simulink model "startSensCompEnv"  (R2021a)
settings: Solver=VariableStepAuto  StartTime=0.0  StopTime=10.0  RelTol=1e-3
undefined symbols (not defined in the file): CubeSatTimeStep, IAU, initCond, km, s, vehicle
libraries: dspmathops x6, sharedtransform x3, aerolibtransform2 x1, aerolibconvert2 x1, aerolibutil x1, aerolibcelestial x1
settings Model: Creator=noraw  LastModifiedBy=noraw

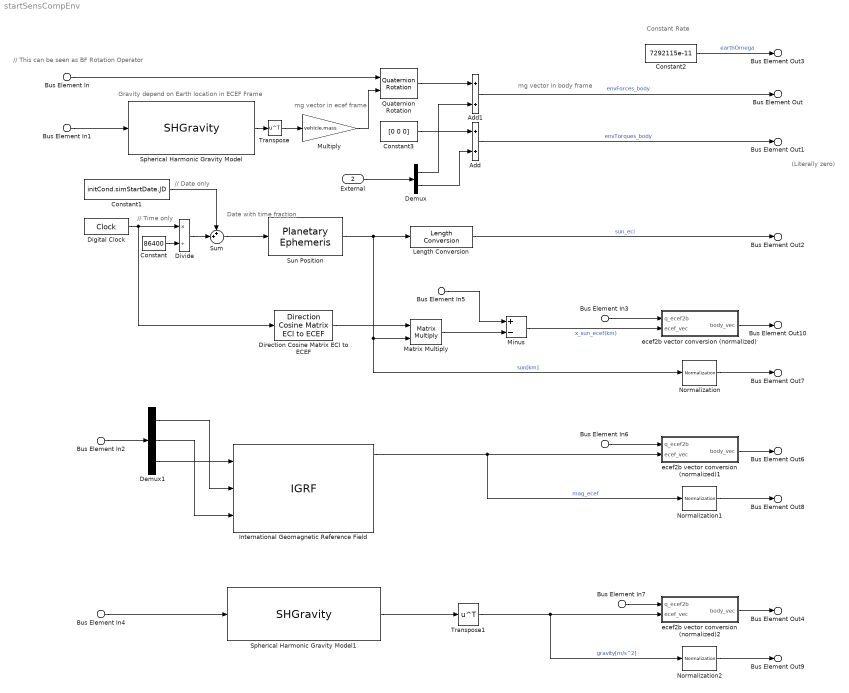
== system startSensCompEnv ==
  note: // Date only
  note: // This can be seen as BF Rotation Operator
  note: Gravity depend on Earth location in ECEF Frame
  note: (Literally zero)
  note: Constant Rate
  note: mg vector in body frame
  note: mg vector in ecef frame
  note: // Time only
  note: Date with
      | time fraction
  Bus Element In{,3,6..7} (4 alike) : Inport  PortName=States  Element=q_ecef2b
  Bus Element In1 : Inport  PortName=States  Element=X_ecef
  Bus Element In4 : Inport  PortName=States  Element=X_ecef
  Bus Element In5 : Inport  PortName=States  Element=X_ecef
  Bus Element In2 : Inport  PortName=States  Element=LatLonAlt
  External : Inport  Port=2
  Add : Sum
  Add1 : Sum
  Constant : Constant  Value=86400
  Constant1 : Constant  Value=initCond.simStartDate.JD
  Constant2 : Constant  Value=7292115e-11
  Constant3 : Constant  Value=[0 0 0]
  Demux : Demux  Outputs=2
  Demux1 : Demux  Outputs=3
  Digital Clock : DigitalClock  SampleTime=CubeSatTimeStep
  Direction Cosine Matrix ECI to ECEF : aerolibtransform2/Direction Cosine Matrix ECI to ECEF  red=IAU-2000/2006  year=2019  month=January  day=4  hour=12  min=0  sec=0  deltaT=Sec  errorflag=Error  extraparamflag=off
      settings: AttributesFormatString=%<red>  SourceProductBaseCode=AE
  Divide : Product  Inputs=*/
  International Geomagnetic Reference Field : IGRF  time_in=off  month=January  day=1  year=2020  sv_out=off
      settings: AttributesFormatString=%<generation>
  Length Conversion : aerolibconvert2/Length Conversion  IU=km  OU=m
  Matrix Multiply : Product  Multiplication=Matrix(*)
  Minus : Sum  Inputs=+-
  Multiply : Gain  Gain=vehicle.mass
  Normalization : dspmathops/Normalization  NormType=Squared 2-norm  Bias=1e-10  NormOver=Each column  Dimension=1  roundingMode=Floor  overflowMode=off  accumDataTypeStr=Inherit: Same as product output  accumLastDataTypeStr=Inherit: Same as product output  outputDataTypeStr=Inherit: Same as product output  outputMin=[]  outputMax=[]  outputLastDataTypeStr=Inherit: Same as product output
  Normalization1 : dspmathops/Normalization  NormType=Squared 2-norm  Bias=1e-10  NormOver=Each column  Dimension=1  roundingMode=Floor  overflowMode=off  accumDataTypeStr=Inherit: Same as product output  accumLastDataTypeStr=Inherit: Same as product output  outputDataTypeStr=Inherit: Same as product output  outputMin=[]  outputMax=[]  outputLastDataTypeStr=Inherit: Same as product output
  Normalization2 : dspmathops/Normalization  NormType=Squared 2-norm  Bias=1e-10  NormOver=Each column  Dimension=1  roundingMode=Floor  overflowMode=off  accumDataTypeStr=Inherit: Same as product output  accumLastDataTypeStr=Inherit: Same as product output  outputDataTypeStr=Inherit: Same as product output  outputMin=[]  outputMax=[]  outputLastDataTypeStr=Inherit: Same as product output
  Quaternion Rotation : aerolibutil/Quaternion Rotation
  Spherical Harmonic Gravity Model : SHGravity  degree=20  datafile='aerogmm2b.mat'
  Spherical Harmonic Gravity Model1 : SHGravity  datafile='aerogmm2b.mat'
  Sum : Sum  Inputs=++|
  Sun Position : aerolibcelestial/Planetary Ephemeris  kmflag=km,km/s  epochflag=Julian date  de=DE421  nCenter=Earth  nTarget=Sun  errorflag=Error  velflag=off
      settings: AttributesFormatString=Ephemeris Data Unavailable  SourceProductName=Aerospace Blockset
  Transpose : Math  Operator=transpose  SignedPower=on  SaturateOnIntegerOverflow=on
  Transpose1 : Math  Operator=transpose  SaturateOnIntegerOverflow=on
  ecef2b vector conversion (normalized) : Subsystem
  ecef2b vector conversion (normalized)1 : Subsystem
  ecef2b vector conversion (normalized)2 : Subsystem
  Bus Element Out : Outport  VectorParamsAs1DForOutWhenUnconnected=off  PortName=Env  Element=envForces_body
  Bus Element Out1 : Outport  VectorParamsAs1DForOutWhenUnconnected=off  PortName=Env  Element=envTorques_body
  Bus Element Out2 : Outport  VectorParamsAs1DForOutWhenUnconnected=off  PortName=Env  Element=x_sun_eci
  Bus Element Out3 : Outport  VectorParamsAs1DForOutWhenUnconnected=off  PortName=Env  Element=earthAngRate
  Bus Element Out10 : Outport  Port=2  PortName=EnvSens  Element=SatFromSun_vec_b
  Bus Element Out6 : Outport  Port=2  PortName=EnvSens  Element=MagOnSat_vec_b
  Bus Element Out4 : Outport  Port=2  PortName=EnvSens  Element=GrvOnSat_vec_b
  Bus Element Out7 : Outport  Port=3  PortName=EnvComp  Element=SatFromSun_vec_f
  Bus Element Out8 : Outport  Port=3  PortName=EnvComp  Element=MagOnSat_vec_f
  Bus Element Out9 : Outport  Port=3  PortName=EnvComp  Element=GrvOnSat_vec_f
  wires:
  Normalization2/1 -> Bus Element Out9/1
  ecef2b vector conversion (normalized)1/1(body_vec) -> Bus Element Out6/1
  Normalization1/1 -> Bus Element Out8/1
  Normalization/1 -> Bus Element Out7/1
  Bus Element In/1 -> Quaternion Rotation/1
  Bus Element In6/1 -> ecef2b vector conversion (normalized)1/1(q_ecef2b)
  Minus/1 -> ecef2b vector conversion (normalized)/2(ecef_vec)  "x_sun_ecef(km)"
  ecef2b vector conversion (normalized)2/1(body_vec) -> Bus Element Out4/1
  International Geomagnetic Reference Field/1 -> Normalization1/1, ecef2b vector conversion (normalized)1/2(ecef_vec)  "mag_ecef"
  Bus Element In7/1 -> ecef2b vector conversion (normalized)2/1(q_ecef2b)
  Demux1/2 -> International Geomagnetic Reference Field/3
  Transpose1/1 -> Normalization2/1, ecef2b vector conversion (normalized)2/2(ecef_vec)  "gravity[m/s^2]"
  Add/1 -> Bus Element Out1/1  "envTorques_body"
  Bus Element In5/1 -> Minus/1
  Divide/1 -> Sum/2
  ecef2b vector conversion (normalized)/1(body_vec) -> Bus Element Out10/1
  Constant1/1 -> Sum/1
  Demux/1 -> Add1/2
  Bus Element In4/1 -> Spherical Harmonic Gravity Model1/1
  Quaternion Rotation/1 -> Add1/1
  Digital Clock/1 -> Direction Cosine Matrix ECI to ECEF/1, Divide/1
  Add1/1 -> Bus Element Out/1  "envForces_body"
  Bus Element In2/1 -> Demux1/1
  Matrix Multiply/1 -> Minus/2
  Direction Cosine Matrix ECI to ECEF/1 -> Matrix Multiply/1
  Demux1/3 -> International Geomagnetic Reference Field/1
  Spherical Harmonic Gravity Model/1 -> Transpose/1
  Bus Element In3/1 -> ecef2b vector conversion (normalized)/1(q_ecef2b)
  External/1 -> Demux/1
  Multiply/1 -> Quaternion Rotation/2
  Transpose/1 -> Multiply/1
  Demux/2 -> Add/2
  Bus Element In1/1 -> Spherical Harmonic Gravity Model/1
  Demux1/1 -> International Geomagnetic Reference Field/2
  Length Conversion/1 -> Bus Element Out2/1  "sun_eci"
  Sun Position/1 -> Length Conversion/1, Matrix Multiply/2, Normalization/1  "sun[km]"
  Spherical Harmonic Gravity Model1/1 -> Transpose1/1
  Sum/1 -> Sun Position/1
  Constant2/1 -> Bus Element Out3/1  "earthOmega"
  Constant3/1 -> Add/1
  Constant/1 -> Divide/2

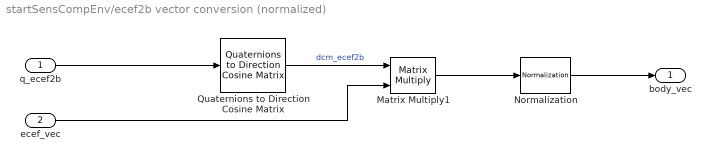
== system startSensCompEnv/ecef2b vector conversion (normalized) ==
  q_ecef2b : Inport
  ecef_vec : Inport  Port=2
  Matrix Multiply1 : Product  Multiplication=Matrix(*)
  Normalization : dspmathops/Normalization  NormType=Squared 2-norm  Bias=1e-10  NormOver=Each column  Dimension=1  roundingMode=Floor  overflowMode=off  accumDataTypeStr=Inherit: Same as product output  accumLastDataTypeStr=Inherit: Same as product output  outputDataTypeStr=Inherit: Same as product output  outputMin=[]  outputMax=[]  outputLastDataTypeStr=Inherit: Same as product output
  Quaternions to Direction Cosine Matrix : sharedtransform/Quaternions to  Direction Cosine Matrix  aMode=aMode
      settings: SourceProductBaseCode=AE,PW,DR,MT,UV,VE
  body_vec : Outport
  wires:
  Quaternions to Direction Cosine Matrix/1 -> Matrix Multiply1/1  "dcm_ecef2b"
  ecef_vec/1 -> Matrix Multiply1/2
  q_ecef2b/1 -> Quaternions to Direction Cosine Matrix/1
  Matrix Multiply1/1 -> Normalization/1
  Normalization/1 -> body_vec/1

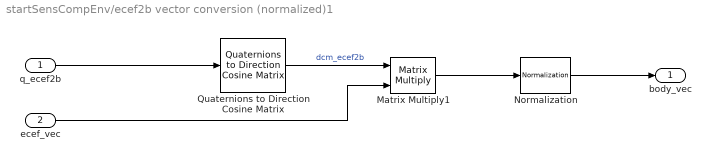
== system startSensCompEnv/ecef2b vector conversion (normalized)1 ==
  q_ecef2b : Inport
  ecef_vec : Inport  Port=2
  Matrix Multiply1 : Product  Multiplication=Matrix(*)
  Normalization : dspmathops/Normalization  NormType=Squared 2-norm  Bias=1e-10  NormOver=Each column  Dimension=1  roundingMode=Floor  overflowMode=off  accumDataTypeStr=Inherit: Same as product output  accumLastDataTypeStr=Inherit: Same as product output  outputDataTypeStr=Inherit: Same as product output  outputMin=[]  outputMax=[]  outputLastDataTypeStr=Inherit: Same as product output
  Quaternions to Direction Cosine Matrix : sharedtransform/Quaternions to  Direction Cosine Matrix  aMode=aMode
      settings: SourceProductBaseCode=AE,PW,DR,MT,UV,VE
  body_vec : Outport
  wires:
  Quaternions to Direction Cosine Matrix/1 -> Matrix Multiply1/1  "dcm_ecef2b"
  ecef_vec/1 -> Matrix Multiply1/2
  q_ecef2b/1 -> Quaternions to Direction Cosine Matrix/1
  Matrix Multiply1/1 -> Normalization/1
  Normalization/1 -> body_vec/1

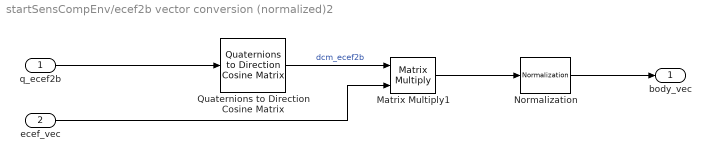
== system startSensCompEnv/ecef2b vector conversion (normalized)2 ==
  q_ecef2b : Inport
  ecef_vec : Inport  Port=2
  Matrix Multiply1 : Product  Multiplication=Matrix(*)
  Normalization : dspmathops/Normalization  NormType=Squared 2-norm  Bias=1e-10  NormOver=Each column  Dimension=1  roundingMode=Floor  overflowMode=off  accumDataTypeStr=Inherit: Same as product output  accumLastDataTypeStr=Inherit: Same as product output  outputDataTypeStr=Inherit: Same as product output  outputMin=[]  outputMax=[]  outputLastDataTypeStr=Inherit: Same as product output
  Quaternions to Direction Cosine Matrix : sharedtransform/Quaternions to  Direction Cosine Matrix  aMode=aMode
      settings: SourceProductBaseCode=AE,PW,DR,MT,UV,VE
  body_vec : Outport
  wires:
  Quaternions to Direction Cosine Matrix/1 -> Matrix Multiply1/1  "dcm_ecef2b"
  ecef_vec/1 -> Matrix Multiply1/2
  q_ecef2b/1 -> Quaternions to Direction Cosine Matrix/1
  Matrix Multiply1/1 -> Normalization/1
  Normalization/1 -> body_vec/1
